simulink model "sim_filterCompare_16b"  (R2016b)
settings: Solver=FixedStepAuto  StartTime=0.0  StopTime=30  FixedStep=1e-3  RelTol=1e-3
undefined symbols (not defined in the file or in its folder): Acc_uDot_mPerScnd2, Acc_vDot_mPerScnd2, Acc_wDot_mPerScnd2, AgVel_p_radPerScnd, AgVel_q_radPerScnd, AgVel_r_radPerScnd
settings Model: Creator=Nu  LastModifiedBy=Nu

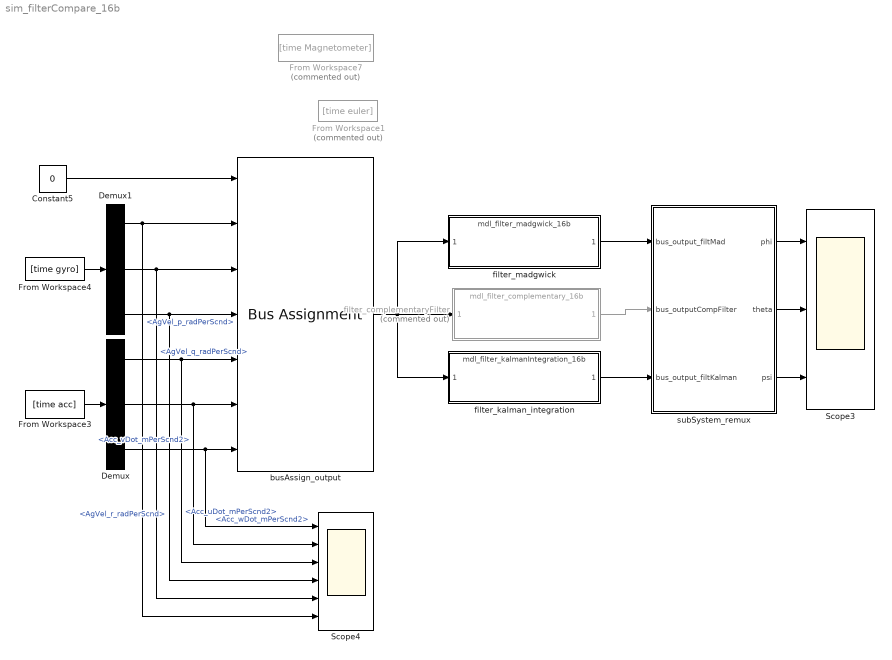
== system sim_filterCompare_16b ==
  Constant5 : Constant  Value=0  OutDataTypeStr=Bus: mdl_output
  Demux : Demux  Outputs=3
  Demux1 : Demux  Outputs=3
  From Workspace1 : FromWorkspace  Commented=on  VariableName=[time euler]  SampleTime=0
  From Workspace3 : FromWorkspace  VariableName=[time acc]  SampleTime=0
  From Workspace4 : FromWorkspace  VariableName=[time gyro]  SampleTime=0
  From Workspace7 : FromWorkspace  Commented=on  VariableName=[time Magnetometer]  SampleTime=0
  Scope3 : Scope  NumInputPorts=3
  Scope4 : Scope  NumInputPorts=6
  busAssign_output : BusAssignment  AssignedSignals=AgVel_p_radPerScnd,AgVel_q_radPerScnd,AgVel_r_radPerScnd,Acc_uDot_mPerScnd2,Acc_vDot_mPerScnd2,Acc_wDot_mPerScnd2
  filter_complementaryFilter : ModelReference  Commented=on  ModelNameDialog=mdl_filter_complementary_16b.slx  SimulationMode=Normal  ModelReferenceVersion=1.30
  filter_kalman_integration : ModelReference  ModelNameDialog=mdl_filter_kalmanIntegration_16b.slx  SimulationMode=Normal  ModelReferenceVersion=1.32
  filter_madgwick : ModelReference  ModelNameDialog=mdl_filter_madgwick_16b.slx  SimulationMode=Normal  ModelReferenceVersion=1.50
  subSystem_remux : Subsystem
  wires:
  From Workspace4/1 -> Demux1/1
  filter_complementaryFilter/1 -> subSystem_remux/2(bus_outputCompFilter)
  filter_kalman_integration/1 -> subSystem_remux/3(bus_output_filtKalman)
  subSystem_remux/1(phi) -> Scope3/1
  subSystem_remux/2(theta) -> Scope3/2
  subSystem_remux/3(psi) -> Scope3/3
  busAssign_output/1 -> filter_madgwick/1, filter_complementaryFilter/1, filter_kalman_integration/1
  Constant5/1 -> busAssign_output/1
  From Workspace3/1 -> Demux/1
  Demux1/3 -> Scope4/4, busAssign_output/4  "<AgVel_r_radPerScnd>"
  Demux1/1 -> Scope4/6, busAssign_output/2  "<AgVel_p_radPerScnd>"
  Demux1/2 -> Scope4/5, busAssign_output/3  "<AgVel_q_radPerScnd>"
  Demux/1 -> Scope4/3, busAssign_output/5  "<Acc_uDot_mPerScnd2>"
  Demux/2 -> Scope4/2, busAssign_output/6  "<Acc_vDot_mPerScnd2>"
  Demux/3 -> Scope4/1, busAssign_output/7  "<Acc_wDot_mPerScnd2>"
  filter_madgwick/1 -> subSystem_remux/1(bus_output_filtMad)

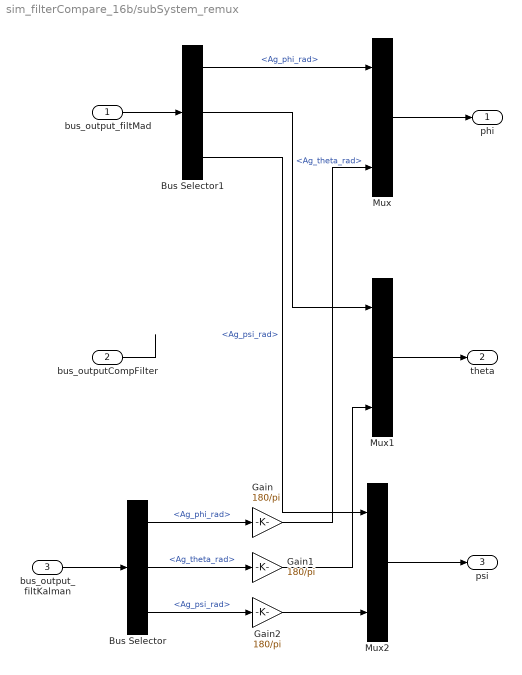
== system sim_filterCompare_16b/subSystem_remux ==
  bus_output_filtMad : Inport
  bus_outputCompFilter : Inport  Port=2
  bus_output_filtKalman : Inport  Port=3
  Bus Selector : BusSelector  OutputSignals=Ag_phi_rad,Ag_theta_rad,Ag_psi_rad
  Bus Selector1 : BusSelector  OutputSignals=Ag_phi_rad,Ag_theta_rad,Ag_psi_rad
  Gain : Gain  Gain=180/pi
  Gain1 : Gain  Gain=180/pi
  Gain2 : Gain  Gain=180/pi
  Mux : Mux  Inputs=3
  Mux1 : Mux  Inputs=3
  Mux2 : Mux  Inputs=3
  phi : Outport
  theta : Outport  Port=2
  psi : Outport  Port=3
  wires:
  ? -> Mux/2
  Bus Selector1/1 -> Mux/1  "<Ag_phi_rad>"
  ? -> Mux1/2
  Mux2/1 -> psi/1
  ? -> Mux2/2
  Bus Selector/3 -> Gain2/1  "<Ag_psi_rad>"
  Mux/1 -> phi/1
  bus_output_filtMad/1 -> Bus Selector1/1
  bus_outputCompFilter/1 -> ?
  Bus Selector1/3 -> Mux2/1  "<Ag_psi_rad>"
  Mux1/1 -> theta/1
  bus_output_filtKalman/1 -> Bus Selector/1
  Bus Selector1/2 -> Mux1/1  "<Ag_theta_rad>"
  Bus Selector/1 -> Gain/1  "<Ag_phi_rad>"
  Bus Selector/2 -> Gain1/1  "<Ag_theta_rad>"
  Gain/1 -> Mux/3
  Gain1/1 -> Mux1/3
  Gain2/1 -> Mux2/3
